simulink model "Anti_lock_break_system_modelling"  (R2020a)
settings: Solver=ode45  StartTime=0.0  StopTime=20  RelTol=1e-3
InitFcn:
  | m = 1200;     % Kg
  | R = 1.25;   % Meter
  | g = 9.81;   % m/s2
  | V0 = 44;    %m/s
  | J = 6;        % kg-m2
settings Model: Creator=Shubham Singh Rathor  LastModifiedBy=Shubham Singh Rathor

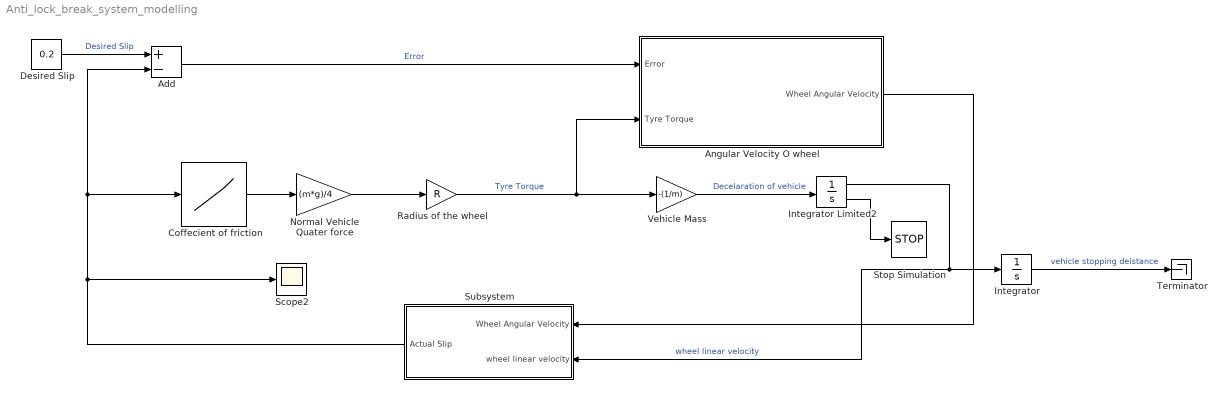
== system Anti_lock_break_system_modelling ==
  Add : Sum  Inputs=+-
  Angular Velocity O wheel : Subsystem
  Coffecient of friction : Lookup_n-D  NumberOfTableDimensions=1  BreakpointsForDimension1=[0:0.05:1]  Table=[0 0.4 0.8 0.97 1 0.98 0.96 0.94 0.92 0.90 0.88 0.855 0.83 0.81 0.79 0.77 0.75 0.73 0.72 0.71 0.70]  InternalRulePriority=Speed  RndMeth=Simplest  InputSameDT=on
  Desired Slip : Constant  Value=0.2
  Integrator : Integrator
  Integrator Limited2 : Integrator  InitialCondition=V0  LimitOutput=on  UpperSaturationLimit=1000  LowerSaturationLimit=0  ShowSaturationPort=on
  Normal Vehicle Quater force : Gain  Gain=(m*g)/4
  Radius of the wheel : Gain  Gain=R
  Scope2 : Scope
  Stop Simulation : Stop
  Subsystem : Subsystem
  Terminator : Terminator
  Vehicle Mass : Gain  Gain=-(1/m)
  wires:
  Desired Slip/1 -> Add/1  "Desired Slip"
  Coffecient of friction/1 -> Normal Vehicle Quater force/1
  Normal Vehicle Quater force/1 -> Radius of the wheel/1
  Radius of the wheel/1 -> Angular Velocity O wheel/2(Tyre Torque), Vehicle Mass/1  "Tyre Torque"
  Vehicle Mass/1 -> Integrator Limited2/1  "Decelaration of vehicle"
  Integrator Limited2/1 -> Integrator/1, Subsystem/2(wheel linear velocity)  "wheel linear velocity"
  Integrator/1 -> Terminator/1  "vehicle stopping deistance"
  Integrator Limited2/2 -> Stop Simulation/1
  Subsystem/1(Actual Slip) -> Add/2, Coffecient of friction/1, Scope2/1
  Add/1 -> Angular Velocity O wheel/1(Error)  "Error"
  Angular Velocity O wheel/1(Wheel Angular Velocity) -> Subsystem/1(Wheel Angular Velocity)

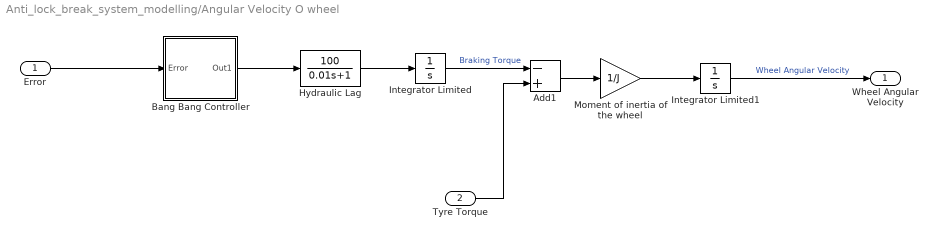
== system Anti_lock_break_system_modelling/Angular Velocity O wheel ==
  Error : Inport
  Tyre Torque : Inport  Port=2
  Add1 : Sum  Inputs=-+
  Bang Bang Controller : Subsystem
  Hydraulic Lag : TransferFcn  Numerator=[100]  Denominator=[0.01 1]
  Integrator Limited : Integrator  LimitOutput=on  UpperSaturationLimit=1000  LowerSaturationLimit=0
  Integrator Limited1 : Integrator  InitialCondition=V0/R  LimitOutput=on  UpperSaturationLimit=1000  LowerSaturationLimit=0
  Moment of inertia of the wheel : Gain  Gain=1/J
  Wheel Angular Velocity : Outport
  wires:
  Error/1 -> Bang Bang Controller/1(Error)
  Tyre Torque/1 -> Add1/2
  Bang Bang Controller/1(Out1) -> Hydraulic Lag/1
  Integrator Limited/1 -> Add1/1  "Braking Torque"
  Hydraulic Lag/1 -> Integrator Limited/1
  Integrator Limited1/1 -> Wheel Angular Velocity/1  "Wheel Angular Velocity"
  Moment of inertia of the wheel/1 -> Integrator Limited1/1
  Add1/1 -> Moment of inertia of the wheel/1

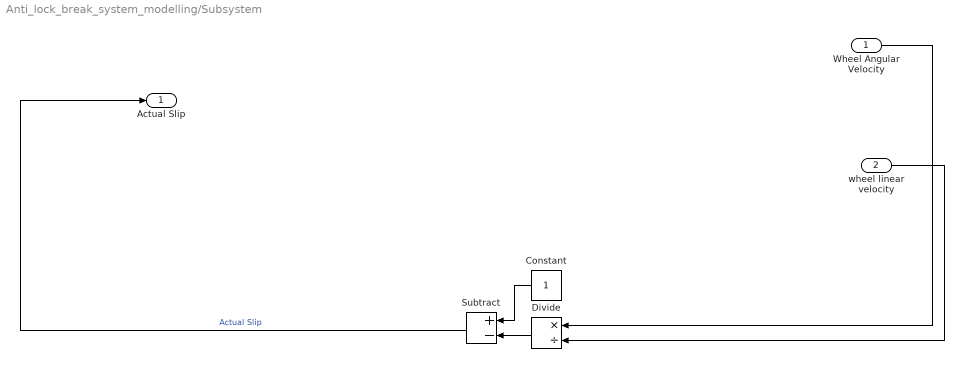
== system Anti_lock_break_system_modelling/Subsystem ==
  Wheel Angular Velocity : Inport
  wheel linear velocity : Inport  Port=2
  Constant : Constant
  Divide : Product  Inputs=*/
  Subtract : Sum  Inputs=+-
  Actual Slip : Outport
  wires:
  Constant/1 -> Subtract/1
  Divide/1 -> Subtract/2
  Subtract/1 -> Actual Slip/1  "Actual Slip"
  Wheel Angular Velocity/1 -> Divide/1
  wheel linear velocity/1 -> Divide/2

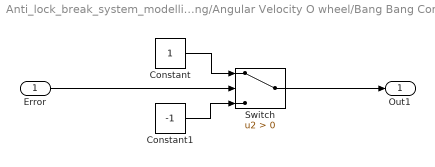
== system Anti_lock_break_system_modelling/Angular Velocity O wheel/Bang Bang Controller ==
  Error : Inport
  Constant : Constant
  Constant1 : Constant  Value=-1
  Switch : Switch  Criteria=u2 > Threshold
  Out1 : Outport
  wires:
  Constant/1 -> Switch/1
  Constant1/1 -> Switch/3
  Switch/1 -> Out1/1
  Error/1 -> Switch/2
